simulink library "aero3D_cl"  (R2020a)
settings: Solver=VariableStepAuto  StartTime=0.0  StopTime=10.0  RelTol=1e-3
undefined symbols (not defined in the file): Veh
libraries: vrlib x1, dynamicPressure_ul x1, alphaY_ul x1, alphaZ_ul x1
settings Model: Creator=John Jr  LastModifiedBy=John Jr

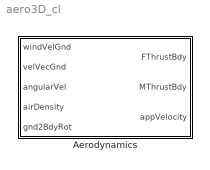
== system aero3D_cl ==
  Aerodynamics : Subsystem  mask{m_m=Veh.motor.motorMass.Value, m_f=Veh.motor.fuelMass.Value, t_b=Veh.motor.burnTime.Value, rM=Veh.motor.position.Value}
      mask prompts: m_m "Total motor mass [kg]"; m_f "Propellant mass [kg]"; t_b "Motor burn time [s]"; rM "Motor position [m]"
      mask DialogControl DescGroupVar Prompt: Rocket Motor Library
      mask DialogControl DescTextVar Prompt: This block models the motor's thrust acting on the vehicle, including rotational effects.
      mask Display:
      | patch([0 1 1 0], [0 0 1 1],[.8 1 1])
      | 
      | port_label('input',1,'\fontname{Cambria Math}windVelGnd','texmode','on')
      | port_label('input',2,'\fontname{Cambria Math}velVecGnd','texmode','on')
      | port_label('input',3,'\fontname{Cambria Math}angularVel','texmode','on')
      | port_label('input',4,'\fontname{Cambria Math}airDensity','texmode','on')
      | port_label('input',5,'\fontname{Cambria Math}gnd2BdyRot','texmode','on')
      | 
      | port_label('output',1,'\fontname{Cambria Math}FAeroBdy','texmode','on')
      | port_label('output',2,'\fontname{Cambria Math}MAeroBdy','texmode','on')
      | port_label('output',3,'\fontname{Cambria Math}appVelocity','texmode','on')

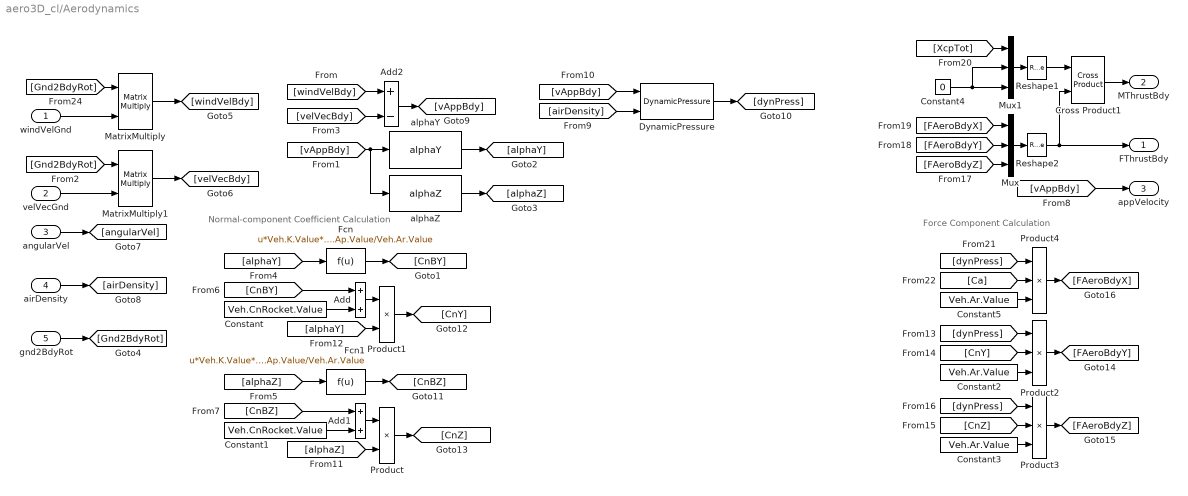
== system aero3D_cl/Aerodynamics ==
  note: Force Component Calculation
  note: Normal-component Coefficient Calculation
  windVelGnd : Inport
  velVecGnd : Inport  Port=2
  angularVel : Inport  Port=3
  airDensity : Inport  Port=4
  gnd2BdyRot : Inport  Port=5
  Add : Sum
  Add1 : Sum
  Add2 : Sum  Inputs=+-
  Constant : Constant  Value=Veh.CnRocket.Value
  Constant1 : Constant  Value=Veh.CnRocket.Value
  Constant2 : Constant  Value=Veh.Ar.Value
  Constant3 : Constant  Value=Veh.Ar.Value
  Constant4 : Constant  Value=0
  Constant5 : Constant  Value=Veh.Ar.Value
  Cross Product1 : vrlib/Utilities/Cross Product
  DynamicPressure : dynamicPressure_ul/DynamicPressure  rho=0
  Fcn : Fcn  Expr=u*Veh.K.Value*Veh.Ap.Value/Veh.Ar.Value
  Fcn1 : Fcn  Expr=u*Veh.K.Value*Veh.Ap.Value/Veh.Ar.Value
  MatrixMultiply : Product  Multiplication=Matrix(*)
  MatrixMultiply1 : Product  Multiplication=Matrix(*)
  Mux : Mux  Inputs=3
  Mux1 : Mux  Inputs=3
  Product : Product
  Product1 : Product
  Product2 : Product  Inputs=3
  Product3 : Product  Inputs=3
  Product4 : Product  Inputs=3
  Reshape1 : Reshape  OutputDimensionality=Column vector (2-D)
  Reshape2 : Reshape  OutputDimensionality=Column vector (2-D)
  alphaY : alphaY_ul/alphaY  SystemSampleTime=-1  Latency=0  AutoFrameSizeCalculation=off
  alphaZ : alphaZ_ul/alphaZ  SystemSampleTime=-1  Latency=0  AutoFrameSizeCalculation=off
  FThrustBdy : Outport  VectorParamsAs1DForOutWhenUnconnected=off
  MThrustBdy : Outport  Port=2  VectorParamsAs1DForOutWhenUnconnected=off
  appVelocity : Outport  Port=3  VectorParamsAs1DForOutWhenUnconnected=off
  wires:
  Cross Product1/1 -> MThrustBdy/1
  Reshape2/1 -> Cross Product1/2, FThrustBdy/1
  gnd2BdyRot/1 -> [Gnd2BdyRot]
  angularVel/1 -> [angularVel]
  airDensity/1 -> [airDensity]
  windVelGnd/1 -> MatrixMultiply/2
  [Gnd2BdyRot] -> MatrixMultiply/1
  velVecGnd/1 -> MatrixMultiply1/2
  [Gnd2BdyRot] -> MatrixMultiply1/1
  MatrixMultiply/1 -> [windVelBdy]
  MatrixMultiply1/1 -> [velVecBdy]
  Add2/1 -> [vAppBdy]
  [windVelBdy] -> Add2/1
  [velVecBdy] -> Add2/2
  [vAppBdy] -> appVelocity/1
  [vAppBdy] -> DynamicPressure/1
  [airDensity] -> DynamicPressure/2
  DynamicPressure/1 -> [dynPress]
  [vAppBdy] -> alphaY/1, alphaZ/1
  alphaY/1 -> [alphaY]
  alphaZ/1 -> [alphaZ]
  [alphaY] -> Fcn/1
  [alphaZ] -> Fcn1/1
  Fcn/1 -> [CnBY]
  Fcn1/1 -> [CnBZ]
  Constant/1 -> Add/2
  [CnBY] -> Add/1
  Constant1/1 -> Add1/2
  [CnBZ] -> Add1/1
  Add1/1 -> Product/1
  [alphaZ] -> Product/2
  Add/1 -> Product1/1
  [alphaY] -> Product1/2
  Product1/1 -> [CnY]
  Product/1 -> [CnZ]
  [dynPress] -> Product2/1
  [CnY] -> Product2/2
  Constant2/1 -> Product2/3
  [dynPress] -> Product3/1
  [CnZ] -> Product3/2
  Constant3/1 -> Product3/3
  Product2/1 -> [FAeroBdyY]
  Product3/1 -> [FAeroBdyZ]
  Mux/1 -> Reshape2/1
  [FAeroBdyY] -> Mux/2
  [FAeroBdyZ] -> Mux/3
  Reshape1/1 -> Cross Product1/1
  Mux1/1 -> Reshape1/1
  Constant4/1 -> Mux1/2, Mux1/3
  [FAeroBdyX] -> Mux/1
  [XcpTot] -> Mux1/1
  Product4/1 -> [FAeroBdyX]
  Constant5/1 -> Product4/3
  [Ca] -> Product4/2
  [dynPress] -> Product4/1
